simulink model "GasExample"  (R2024a)
settings: Solver=VariableStepAuto  StartTime=0.0  StopTime=100  RelTol=1e-3
libraries: Bibliothek_FHDO_V1 x8
settings Model: Creator=goessling  LastModifiedBy=goessling

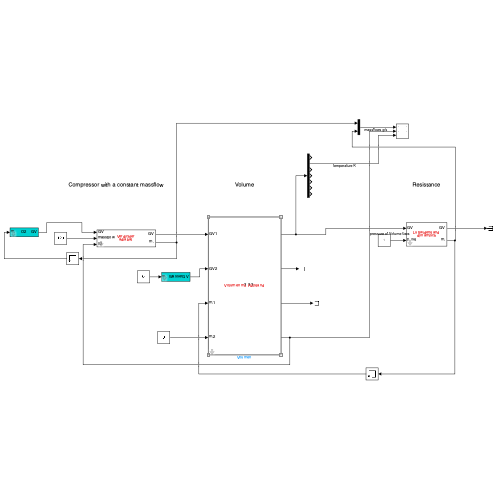
[thumbnail: Simulink's stored preview of the top-level diagram]
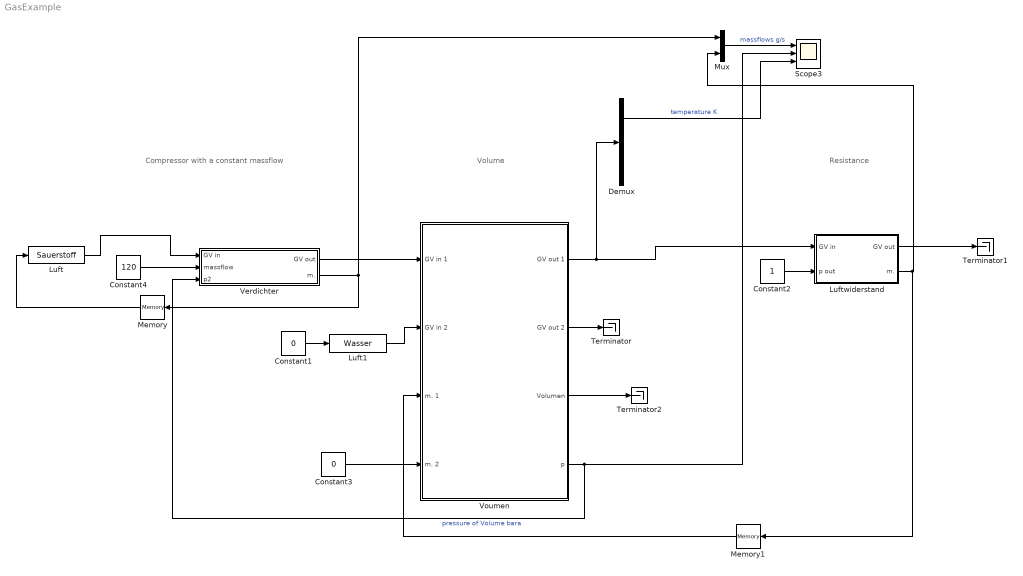
== system GasExample ==
  note: Compressor with a constant massflow
  note: Volume
  note: Resistance
  Constant1 : Constant  Value=0
  Constant2 : Constant
  Constant3 : Constant  Value=0
  Constant4 : Constant  Value=120
  Demux : Demux  Outputs=7
  Luft : Bibliothek_FHDO_V1/Sauerstoff  p=1  T=25
      link override x: Value=[0 0 0.23 0.77]
  Luft1 : Bibliothek_FHDO_V1/Wasser  p=1  T=25
  Luftwiderstand : Subsystem  mask{V_fac=0.012, dp_fac=0.03, exp=1}
      mask prompts: V_fac "Volumenstrom"; dp_fac "Druckverlust"; exp "Verlauf"
      mask Display:
      | color('red')
      | disp('Luftwiderstand\n dynamisch')
      | 
      | color('black')
      | port_label('input', 1, 'GV')
      | port_label('input', 2, 'p out')
      | 
      | port_label('output', 1, 'GV')
      | port_label('output', 2, 'm.')
  Memory : Memory
  Memory1 : Memory
  Mux : Mux  Inputs=2
  Scope3 : Scope  NumInputPorts=3
  Terminator : Terminator
  Terminator1 : Terminator
  Terminator2 : Terminator
  Verdichter : Subsystem  mask{eta_f=0.7}
      mask prompts: eta_f "Wirkungsgrad der Verdichtung"
      mask Display:
      | color('red')
      | disp('Verdichter\nadiabat')
      | 
      | color('black')
      | port_label('input', 1, 'GV')
      | port_label('input', 2, 'massflow')
      | port_label('input', 3, 'p2')
      | 
      | port_label('output', 1, 'GV')
      | port_label('output', 2, 'm.')
  Voumen : Subsystem  mask{V=1, p_start=1, T_start=25, x_start=[0.1 0.9 0 0]}
      mask prompts: V "Volumen [m^3]"; p_start "p [bar]"; T_start "T [°C]"; x_start "x"
      mask Display:
      | color('red')
      | disp(['Volumen mit Füllstand'])
      | 
      | color('black')
      | port_label('input', 1, 'GV1')
      | port_label('input', 2, 'GV2')
      | port_label('input', 3, 'm.1')
      | port_label('input', 4, 'm.2')
      | port_label('input', 5, 'm.unten')
      | 
      | port_label('output', 1, 'GV1')
      | port_label('output', 2, 'GV2')
      | port_label('output', 3, 'V')
      | port_label('output', 4, 'p')
      | port_label('output', 5, 'Fuellstand')
      | port_label('output', 6, 'Liquid out')
  wires:
  Luft/1 -> Verdichter/1(GV in)
  Constant1/1 -> Luft1/1
  Luft1/1 -> Voumen/2(GV in 2)
  Memory/1 -> Luft/1
  Memory1/1 -> Voumen/3(m. 1)
  Constant3/1 -> Voumen/4(m. 2)
  Voumen/3(Volumen) -> Terminator2/1
  Voumen/4(p) -> Scope3/2, Verdichter/3(p2)  "pressure of Volume bara"
  Voumen/1(GV out 1) -> Demux/1, Luftwiderstand/1(GV in)
  Verdichter/1(GV out) -> Voumen/1(GV in 1)
  Verdichter/2(m.) -> Memory/1, Mux/1
  Constant2/1 -> Luftwiderstand/2(p out)
  Luftwiderstand/2(m.) -> Memory1/1, Mux/2
  Mux/1 -> Scope3/1  "massflows g/s"
  Voumen/2(GV out 2) -> Terminator/1
  Luftwiderstand/1(GV out) -> Terminator1/1
  Constant4/1 -> Verdichter/2(massflow)
  Demux/2 -> Scope3/3  "temperature K"

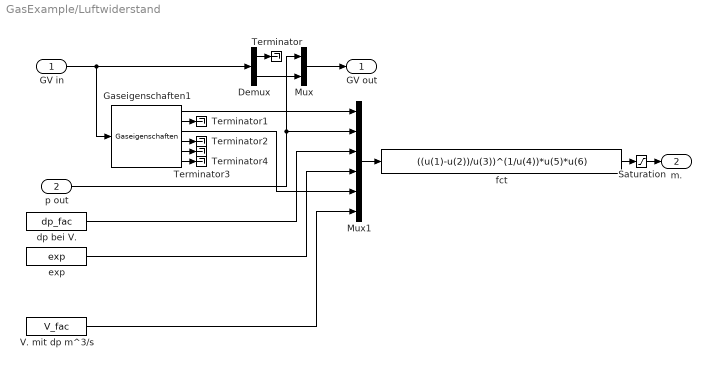
== system GasExample/Luftwiderstand ==
  GV in : Inport
  p out : Inport  Port=2
  Demux : Demux  Outputs=[1 6]
  Gaseigenschaften1 : Bibliothek_FHDO_V1/Gaseigenschaften  SystemSampleTime=-1  VariantActivationTime=update diagram  AllowFlexibleInterface=on  Latency=0  AutoFrameSizeCalculation=off
  Mux : Mux  Inputs=2
  Mux1 : Mux  Inputs=6
  Saturation : Saturate  UpperLimit=inf  LowerLimit=eps
  Terminator{,1..4} (5 alike) : Terminator
  V. mit dp m^3/s : Constant  Value=V_fac
  dp bei V. : Constant  Value=dp_fac
  exp : Constant  Value=exp
  fct : Fcn  Expr=((u(1)-u(2))/u(3))^(1/u(4))*u(5)*u(6)
  GV out : Outport
  m. : Outport  Port=2
  wires:
  Gaseigenschaften1/6 -> Terminator4/1
  Saturation/1 -> m./1
  Gaseigenschaften1/5 -> Terminator3/1
  Gaseigenschaften1/4 -> Terminator2/1
  Gaseigenschaften1/2 -> Terminator1/1
  V. mit dp m^3/s/1 -> Mux1/6
  Gaseigenschaften1/3 -> Mux1/5
  exp/1 -> Mux1/4
  dp bei V./1 -> Mux1/3
  fct/1 -> Saturation/1
  Mux1/1 -> fct/1
  Gaseigenschaften1/1 -> Mux1/1
  Demux/1 -> Terminator/1
  Demux/2 -> Mux/2
  p out/1 -> Mux1/2, Mux/1
  Mux/1 -> GV out/1
  GV in/1 -> Gaseigenschaften1/1, Demux/1

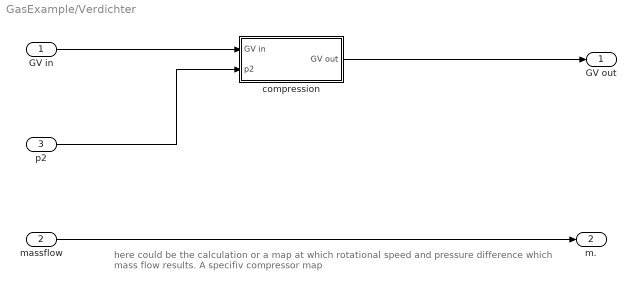
== system GasExample/Verdichter ==
  note: here could be the calculation or a map at which rotational speed and pressure difference which mass flow results. A specifiv compressor map
  GV in : Inport
  massflow : Inport  Port=2
  p2 : Inport  Port=3
  compression : Subsystem
  GV out : Outport
  m. : Outport  Port=2
  wires:
  compression/1(GV out) -> GV out/1
  p2/1 -> compression/2(p2)
  GV in/1 -> compression/1(GV in)
  massflow/1 -> m./1

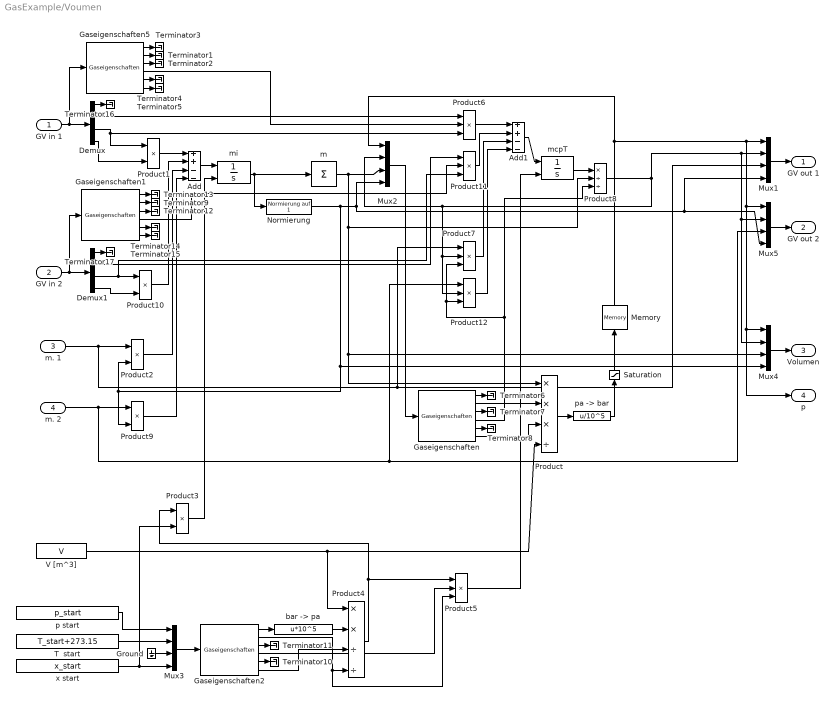
== system GasExample/Voumen ==
  GV in 1 : Inport
  GV in 2 : Inport  Port=2
  m. 1 : Inport  Port=3
  m. 2 : Inport  Port=4
  Add : Sum  Inputs=++--
  Add1 : Sum  Inputs=++--  SampleTime=.01
  Demux : Demux  Outputs=[1 1 1 4]
  Demux1 : Demux  Outputs=[1 1 1 4]
  Gaseigenschaften{,1..2,5} (4 alike) : Bibliothek_FHDO_V1/Gaseigenschaften  SystemSampleTime=-1  VariantActivationTime=update diagram  AllowFlexibleInterface=on  Latency=0  AutoFrameSizeCalculation=off
  Ground : Ground
  Memory : Memory  InitialCondition=p_start
  Mux{1..5} (5 alike) : Mux
  Normierung : Bibliothek_FHDO_V1/Sauerstoff/Normierung auf 1  SystemSampleTime=-1  VariantActivationTime=update diagram  AllowFlexibleInterface=on  Latency=0  AutoFrameSizeCalculation=off
  Product : Product  Inputs=***/  RndMeth=Zero
  Product{1..3,9..10} (5 alike) : Product  RndMeth=Zero
  Product{5..7,11..12} (5 alike) : Product  Inputs=3  RndMeth=Zero
  Product4 : Product  Inputs=**//  RndMeth=Zero
  Product8 : Product  Inputs=*//  RndMeth=Zero
  Saturation : Saturate  UpperLimit=inf  LowerLimit=1
  T  start : Constant  Value=T_start+273.15
  Terminator{1..17} (17 alike) : Terminator
  V [m^3] : Constant  Value=V
  "bar -> pa" : Fcn  Expr=u*10^5
  m : Sum  Inputs=+
  mcpT : Integrator  InitialConditionSource=external  InitialCondition=[0 0 0 0 0 0 .21 .79]*1293
  mi : Integrator  InitialConditionSource=external  InitialCondition=[0 0 0 0 0 0 .21 .79]*1293
  p start : Constant  Value=p_start
  "pa -> bar" : Fcn  Expr=u/10^5
  x start : Constant  Value=x_start
  GV out 1 : Outport
  GV out 2 : Outport  Port=2
  Volumen : Outport  Port=3
  p : Outport  Port=4
  wires:
  GV in 1/1 -> Gaseigenschaften5/1, Demux/1
  Demux/3 -> Product1/1, Product6/3
  Demux/2 -> Product6/1
  Demux/4 -> Product1/2
  Gaseigenschaften/1 -> Terminator6/1
  Gaseigenschaften/4 -> Product8/3, Product7/3, Product12/3
  Product1/1 -> Add/1
  m. 1/1 -> Product2/1, Product7/1, Mux1/3
  mi/1 -> Normierung/1, m/1
  Normierung/1 -> Mux2/4, Mux1/4, Mux5/4, Mux4/4, Product2/2, Product9/2
  Product2/1 -> Add/3
  Add/1 -> mi/1
  m/1 -> Mux2/3, Product8/2, Product/1, Mux4/3
  Mux2/1 -> Gaseigenschaften/1
  Gaseigenschaften5/1 -> Terminator3/1
  Gaseigenschaften5/4 -> Product6/2
  Gaseigenschaften/6 -> Product/3
  Gaseigenschaften/2 -> Product/2
  V [m^3]/1 -> Product4/1, Product/4
  Product/1 -> "pa -> bar"/1
  Mux1/1 -> GV out 1/1
  Gaseigenschaften5/2 -> Terminator1/1
  Gaseigenschaften5/3 -> Terminator2/1
  Gaseigenschaften5/5 -> Terminator4/1
  Gaseigenschaften5/6 -> Terminator5/1
  Gaseigenschaften/3 -> Terminator7/1
  Gaseigenschaften/5 -> Terminator8/1
  "pa -> bar"/1 -> Saturation/1
  x start/1 -> Mux3/4, Product3/2
  Ground/1 -> Mux3/3
  p start/1 -> Mux3/1
  T  start/1 -> Mux3/2
  Mux3/1 -> Gaseigenschaften2/1
  Gaseigenschaften2/1 -> "bar -> pa"/1
  "bar -> pa"/1 -> Product4/2
  Gaseigenschaften2/6 -> Product4/3
  Gaseigenschaften2/2 -> Product4/4, Product5/3
  Gaseigenschaften2/3 -> Terminator11/1
  Gaseigenschaften2/4 -> Product5/2
  Gaseigenschaften2/5 -> Terminator10/1
  Product4/1 -> Product5/1, Product3/1
  Product3/1 -> mi/2
  Product5/1 -> mcpT/2
  Product6/1 -> Add1/1
  Add1/1 -> mcpT/1
  mcpT/1 -> Product8/1
  Product8/1 -> Mux2/2, Product7/2, Product12/2, Mux1/2, Mux4/2, Mux5/2
  Product7/1 -> Add1/3
  m. 2/1 -> Product9/1, Mux5/3, Product12/1
  Product9/1 -> Add/4
  Mux5/1 -> GV out 2/1
  GV in 2/1 -> Gaseigenschaften1/1, Demux1/1
  Gaseigenschaften1/1 -> Terminator13/1
  Gaseigenschaften1/2 -> Terminator9/1
  Gaseigenschaften1/3 -> Terminator12/1
  Gaseigenschaften1/5 -> Terminator14/1
  Gaseigenschaften1/6 -> Terminator15/1
  Demux/1 -> Terminator16/1
  Demux1/1 -> Terminator17/1
  Demux1/3 -> Product10/1, Product11/3
  Demux1/4 -> Product10/2
  Product10/1 -> Add/2
  Product11/1 -> Add1/2
  Product12/1 -> Add1/4
  Gaseigenschaften1/4 -> Product11/2
  Demux1/2 -> Product11/1
  Memory/1 -> Mux1/1, Mux5/1, Mux4/1, p/1, Mux2/1
  Saturation/1 -> Memory/1
  Mux4/1 -> Volumen/1

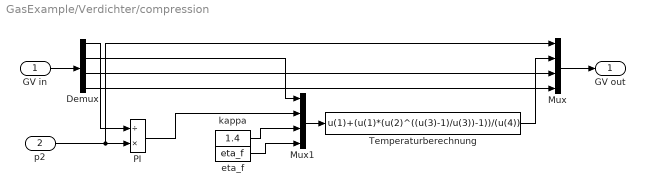
== system GasExample/Verdichter/compression ==
  GV in : Inport
  p2 : Inport  Port=2
  Demux : Demux  Outputs=[1 1 1 4]
  Mux : Mux
  Mux1 : Mux
  PI : Product  Inputs=/*  RndMeth=Zero
  Temperaturberechnung : Fcn  Expr=u(1)+(u(1)*(u(2)^((u(3)-1)/u(3))-1))/(u(4))
  eta_f : Constant  Value=eta_f
  kappa : Constant  Value=1.4
  GV out : Outport
  wires:
  eta_f/1 -> Mux1/4
  kappa/1 -> Mux1/3
  Demux/2 -> Mux1/1
  Mux1/1 -> Temperaturberechnung/1
  Temperaturberechnung/1 -> Mux/2
  Demux/4 -> Mux/4
  Demux/3 -> Mux/3
  Mux/1 -> GV out/1
  PI/1 -> Mux1/2
  p2/1 -> Mux/1, PI/2
  Demux/1 -> PI/1
  GV in/1 -> Demux/1
